simulink model "gain_ex3"  (R2020b)
settings: Solver=VariableStepAuto  StartTime=0.0  StopTime=10.0  RelTol=1e-3
settings Model: Creator=Lenovo  LastModifiedBy=Lenovo

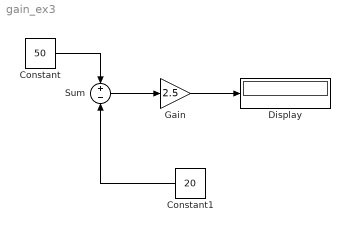
== system gain_ex3 ==
  Constant : Constant  Value=50
  Constant1 : Constant  Value=20
  Display : Display
  Gain : Gain  Gain=2.5
  Sum : Sum  Inputs=+-
  wires:
  Constant/1 -> Sum/1
  Sum/1 -> Gain/1
  Gain/1 -> Display/1
  Constant1/1 -> Sum/2
